simulink model "PNEU_PID"  (R2022b)
settings: Solver=ode14x  StartTime=0.0  StopTime=10  FixedStep=1e-3  RelTol=1e-3
values from neighbouring files (symbols this model uses):
  Aa = 6.91e-4    (= 0.000691)    [PNEU_PARAMETROS.m]
  Ab = 8.94e-4    (= 0.000894)    [PNEU_PARAMETROS.m]
  GuA0 = 3.2e3    (= 3200)    [PNEU_PARAMETROS.m]
  GuB0 = 3.2e3    (= 3200)    [PNEU_PARAMETROS.m]
  ka = 36    [PNEU_PARAMETROS.m]
  kd = K    [PID_FMIN_WeightedError.m]    (also in PID_FMIN_WeightedError_Main.m = 0.1)
  ki = (z1*z2)*kd    [PID_FMIN_WeightedError.m]    (also in PID_FMIN_WeightedError_Main.m = 6)
  kp = (z1 + z2)*kd    [PID_FMIN_WeightedError.m]    (also in PID_FMIN_WeightedError_Main.m = 1.6)
  M = 2.7    [PNEU_PARAMETROS.m]
  PA0 = 4.97    [PNEU_PARAMETROS.m]
  PB0 = 5.61    [PNEU_PARAMETROS.m]
  R = 8.314e-5    (= 8.314e-05)    [PNEU_PARAMETROS.m]
  ta = 0.112    [PNEU_PARAMETROS.m]
  TA0 = 293.15    [PNEU_PARAMETROS.m]
  tb = 0.104    [PNEU_PARAMETROS.m]
  TB0 = 293.15    [PNEU_PARAMETROS.m]
  VA0 = 0.2*Aa    (= 0.0001382)    [PNEU_PARAMETROS.m]
  VB0 = 0.2*Ab    (= 0.0001788)    [PNEU_PARAMETROS.m]
  y = sim("PNEU_PID.slx")    [PID_FMIN_WeightedError.m]    (also in PNEU_PARAMETROS.m = 1.4)
libraries: slpidlib x1
settings Model: Creator=AndreiaOliveira  LastModifiedBy=AndreiaOliveira

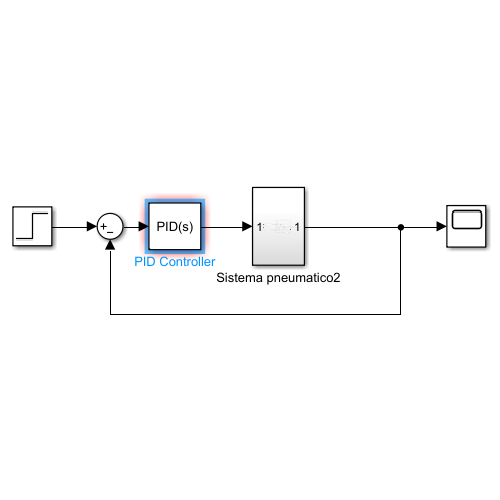
[thumbnail: Simulink's stored preview of the top-level diagram]
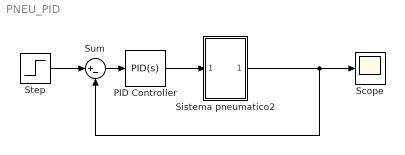
== system PNEU_PID ==
  PID Controller : slpidlib/PID Controller  Controller=PID  Form=Parallel  TimeDomain=Continuous-time  UseExternalTs=off  SampleTime=-1  IntegratorMethod=Forward Euler  FilterMethod=Forward Euler  ControllerParametersSource=internal  P=kp  I=ki  UseKiTs=off  D=kd  N=100  UseFilter=on  TunerSelectOption=Transfer Function Based (PID Tuner App)  InitialConditionSource=internal  InitialConditionForIntegrator=0  InitialConditionForFilter=0  DifferentiatorICPrevScaledInput=0  ExternalReset=none  TrackingMode=off  Kt=1  LimitOutput=off  SatLimitsSource=internal  UpperSaturationLimit=inf  LowerSaturationLimit=-inf  LinearizeAsGain=on  AntiWindupMode=none  Kb=1  LimitIntegrator=off  UpperIntegratorSaturationLimit=inf  LowerIntegratorSaturationLimit=-inf  POutMin=[]  POutMax=[]  IOutMin=[]  IOutMax=[]  DOutMin=[]  DOutMax=[]  NOutMin=[]  NOutMax=[]  SumOutMin=[]  SumOutMax=[]  SaturationOutMin=[]  SaturationOutMax=[]  PParamMin=[]  PParamMax=[]  IParamMin=[]  IParamMax=[]  DParamMin=[]  DParamMax=[]  NParamMin=[]  NParamMax=[]  KbParamMin=[]  KbParamMax=[]  KtParamMin=[]  KtParamMax=[]  KbOutMin=[]  KbOutMax=[]  KtOutMin=[]  KtOutMax=[]  IntegratorOutMin=[]  IntegratorOutMax=[]  FilterOutMin=[]  FilterOutMax=[]  SumI1OutMin=[]  SumI1OutMax=[]  SumI2OutMin=[]  SumI2OutMax=[]  SumI3OutMin=[]  SumI3OutMax=[]  SumI4OutMin=[]  SumI4OutMax=[]  SumDOutMin=[]  SumDOutMax=[]  DifferentiatorOutMin=[]  DifferentiatorOutMax=[]  FilterDiffOutCoefMin=[]  FilterDiffOutCoefMax=[]  ReciprocalOutMin=[]  ReciprocalOutMax=[]  SumDenOutMin=[]  SumDenOutMax=[]  SumNumOutMin=[]  SumNumOutMax=[]  DivideOutMin=[]  DivideOutMax=[]  UdiffTsProdOutMin=[]  UdiffTsProdOutMax=[]  NTsProdOutMin=[]  NTsProdOutMax=[]  UintegralTsProdOutMin=[]  UintegralTsProdOutMax=[]  UngainTsProdOutMin=[]  UngainTsProdOutMax=[]  ClampingZeroOutDataTypeStr=Inherit: Inherit via back propagation  ClampingZeroOutMin=[]  ClampingZeroOutMax=[]  FilterDenConstantOutDataTypeStr=Inherit: Inherit via back propagation  FilterDenConstantOutMin=[]  FilterDenConstantOutMax=[]  PCopyOutDataTypeStr=Inherit: Inherit via back propagation  PCopyOutMin=[]  PCopyOutMax=[]  NCopyOutDataTypeStr=Inherit: Inherit via back propagation  NCopyOutMin=[]  NCopyOutMax=[]  IntegratorContinuousStateAttributes=''  IntegratorStateMustResolveToSignalObject=off  IntegratorRTWStateStorageClass=Auto  FilterContinuousStateAttributes=''  FilterStateMustResolveToSignalObject=off  FilterRTWStateStorageClass=Auto  ParallelPVariant=InternalParameters  IdealPVariant=Disabled  IVariant=InternalParameters  DVariant=InternalParameters  IntegratorVariant=Continuous  SatVariant=Disabled  AWVariant=Passthrough  PCopyVariant=Disabled  TRVariant=Disabled  FdbkBlocksVariant=Forward  IdealPFdbkVariant=Disabled  SatFdbkVariant=Disabled  DerivativeFilterVariant=ContFilter  NVariant=InternalParameters  NCopyVariant=Disabled  FilterICVariant=InternalICsFilter  IntegratorICVariant=InternalICs  ExternalResetVariant=Disabled  TRSumVariant=Passthrough  SumFdbkVariant=Disabled  SumVariant=Sum_PID  TsampFilterVariant=InternalTs  TsampNgainVariant=Passthrough  TsampIntegralVariant=Passthrough  ExternalSaturationOutDataTypeStr=Inherit: Same as second input
  Scope : Scope
  Sistema pneumatico2 : Subsystem
  Step : Step  SampleTime=0
  Sum : Sum  Inputs=|+-
  wires:
  Sistema pneumatico2/1(Out1) -> Sum/2, Scope/1
  Sum/1 -> PID Controller/1
  PID Controller/1 -> Sistema pneumatico2/1(In1)
  Step/1 -> Sum/1

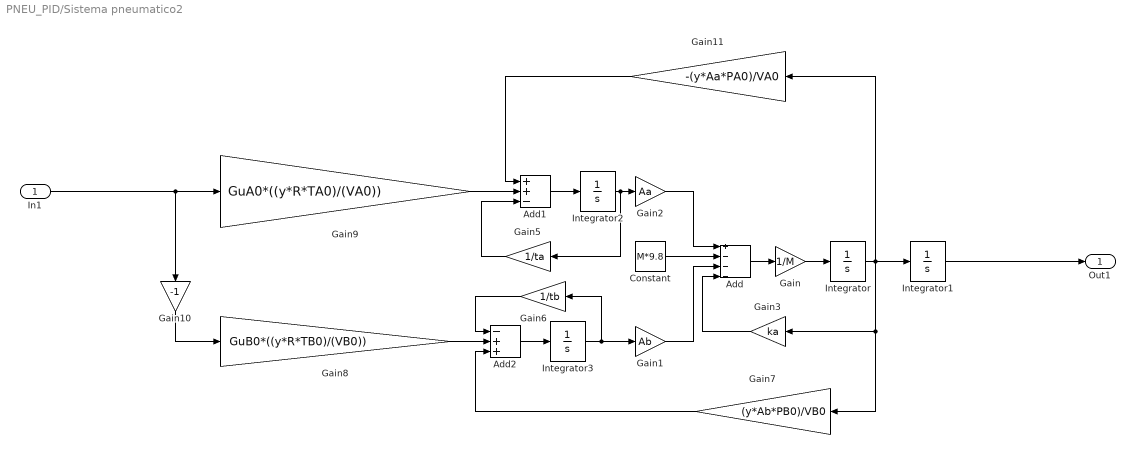
== system PNEU_PID/Sistema pneumatico2 ==
  In1 : Inport
  Add : Sum  Inputs=+---
  Add1 : Sum  Inputs=++-
  Add2 : Sum  Inputs=-++
  Constant : Constant  Value=M*9.8
  Gain : Gain  Gain=1/M
  Gain1 : Gain  Gain=Ab
  Gain10 : Gain  Gain=-1
  Gain11 : Gain  Gain=-(y*Aa*PA0)/VA0
  Gain2 : Gain  Gain=Aa
  Gain3 : Gain  Gain=ka
  Gain5 : Gain  Gain=1/ta
  Gain6 : Gain  Gain=1/tb
  Gain7 : Gain  Gain=(y*Ab*PB0)/VB0
  Gain8 : Gain  Gain=GuB0*((y*R*TB0)/(VB0))
  Gain9 : Gain  Gain=GuA0*((y*R*TA0)/(VA0))
  Integrator{,1..3} (4 alike) : Integrator
  Out1 : Outport
  wires:
  Gain8/1 -> Add2/2
  Integrator3/1 -> Gain6/1, Gain1/1
  In1/1 -> Gain9/1, Gain10/1
  Gain6/1 -> Add2/1
  Gain3/1 -> Add/4
  Gain5/1 -> Add1/3
  Integrator2/1 -> Gain5/1, Gain2/1
  Gain10/1 -> Gain8/1
  Gain2/1 -> Add/1
  Constant/1 -> Add/2
  Gain1/1 -> Add/3
  Add1/1 -> Integrator2/1
  Add2/1 -> Integrator3/1
  Gain9/1 -> Add1/2
  Integrator/1 -> Integrator1/1, Gain11/1, Gain7/1, Gain3/1
  Gain/1 -> Integrator/1
  Add/1 -> Gain/1
  Integrator1/1 -> Out1/1
  Gain7/1 -> Add2/3
  Gain11/1 -> Add1/1
